simulink library "tools"  (R2015b)
settings: Solver=ode1  StartTime=0.0  StopTime=Inf  FixedStep=0.001  RelTol=1e-3
PostLoadFcn:
  | , if any(exist('dsrtsu_mdlpostloadfcn', 'file') == [2, 3, 6]), try dsrtsu_mdlpostloadfcn('Execute', bdroot); catch fprintf('Error in PostLoadFcn (dsrtsu_mdlpostloadfcn) for model "%s":\n %s\n', bdroot, lasterr); end, end,
libraries: tools x3, dspswit3 x2
settings Model: DSRTSU_INTERNAL_RTI_VER=460  DSRTSU_INTERNAL_RTI_TYPE=rti1401  DSRTSU_INTERNAL_RTIFPGA=50  Creator=luis  LastModifiedBy=luis
settings OptimizationCC: BlockReduction=off  OptimizeBlockIOStorage=off  BufferReuse=off  GlobalBufferReuse=off  ExpressionFolding=off  LocalBlockOutputs=off
settings HardwareCC: ProdEndianess=BigEndian  ProdWordSize=32  ProdHWDeviceType=Generic->Custom  TargetIntDivRoundTo=Zero  TargetEndianess=BigEndian  TargetHWDeviceType=Generic->Custom
settings RTWCC: SystemTargetFile=rti1401.tlc  MakeCommand=make_rti  TemplateMakefile=rti1401.tmf  Description=dSPACE DS1401 Hardware Platform
settings STFCustomTargetCC: ParMdlRefBuildCompliant=on  ConcurrentExecutionCompliant=off  GeneratePreprocessorConditionals=Use local settings  MatFileLogging=on  CPPClassGenCompliant=off  SystemTargetFile=rti1401.tlc
settings GRTTargetCC: CompOptLevelCompliant=off  ConcurrentExecutionCompliant=off  CombineOutputUpdateFcns=off  CPPClassGenCompliant=off  GRTInterface=on  UseToolchainInfoCompliant=off  ExtModeMexFile=noextcomm

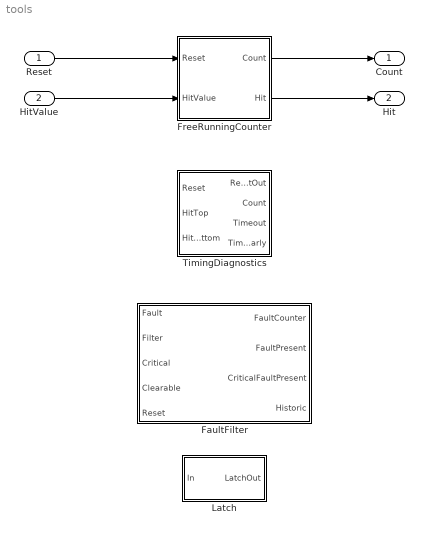
== system tools ==
  Reset : Inport
  HitValue : Inport  Port=2
  FaultFilter : Subsystem
  FreeRunningCounter : Subsystem
  Latch : Subsystem
  TimingDiagnostics : Subsystem
  Count : Outport
  Hit : Outport  Port=2
  wires:
  Reset/1 -> FreeRunningCounter/1(Reset)
  HitValue/1 -> FreeRunningCounter/2(HitValue)
  FreeRunningCounter/1(Count) -> Count/1
  FreeRunningCounter/2(Hit) -> Hit/1

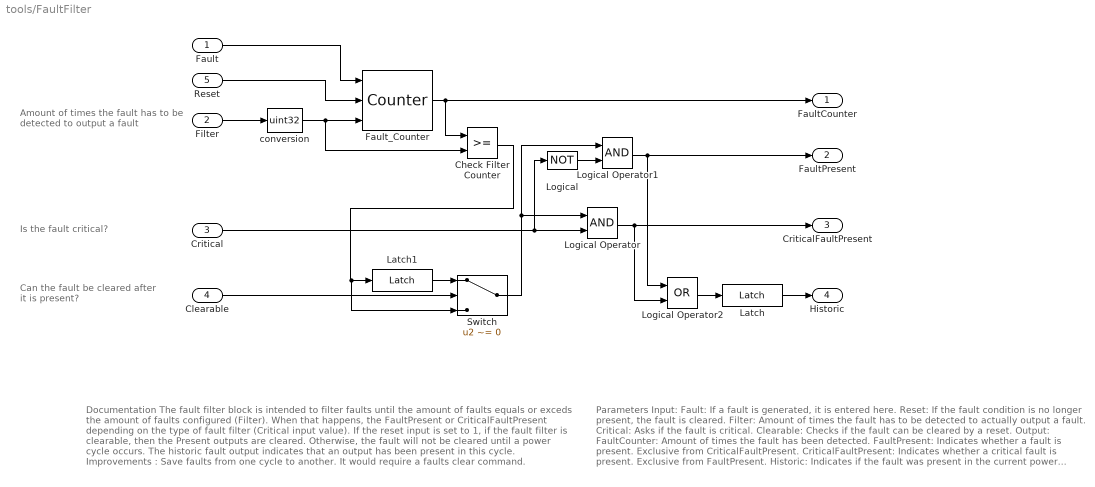
== system tools/FaultFilter ==
  note: Parameters
      | Input:
      | Fault: If a fault is generated, it is entered here.
      | Reset: If the fault condition is no longer present, the fault is cleared.
      | Filter: Amount of times the fault has to be detected to actually output a fault.
      | Critical: Asks if the fault is critical.
      | Clearable: Checks if the fault can be cleared by a reset.
      |
      | Output:
      | FaultCounter: Amount of times the fault has been detected.
      | FaultPresent: Indicates whether a fault is present. Exclusive from CriticalFaultPresent.
      | CriticalFaultPresent: Indicates whether a critical fault is present. Exclusive from FaultPresent.
      | Historic: Indicates if the fault was present in the current power cycle.
  note: Can the fault be cleared
      | after it is present?
  note: Is the fault critical?
  note: Amount of times the fault
      | has to be detected to output a fault
  note: Documentation
      | The fault filter block is intended to filter faults until the amount of faults equals or exceds the amount of faults configured (Filter). When that happens, the FaultPresent or CriticalFaultPresent depending on the type of fault filter (Critical input value). If the reset input is set to 1, if the fault filter is clearable, then the Present outputs are cleared.
      | Otherwise, the fault will not be cleared until a power cycle occurs.
      | The historic fault output indicates that an output has been present in this cycle.
      | Improvements : Save faults from one cycle to another. It would require a faults clear command.
  Fault : Inport
  Filter : Inport  Port=2
  Critical : Inport  Port=3
  Clearable : Inport  Port=4
  Reset : Inport  Port=5
  Check Filter Counter : RelationalOperator  OutDataTypeStr=boolean
  Fault_Counter : dspswit3/Counter  Direction=Up  CountEvent=Rising edge  CounterSize=Specify via input port  MaxCount=255  InitialCount=0  Output=Count  HitValue=32  ResetInput=on  SamplesPerFrame=1  Ts=-1  CntDtype=double  HitDtype=Logical
  Latch : tools/Latch
  Latch1 : tools/Latch
  Logical : Logic  Operator=NOT  AllPortsSameDT=off  OutDataTypeStr=boolean
  Logical Operator : Logic  AllPortsSameDT=off  OutDataTypeStr=boolean
  Logical Operator1 : Logic  AllPortsSameDT=off  OutDataTypeStr=boolean
  Logical Operator2 : Logic  Operator=OR  AllPortsSameDT=off  OutDataTypeStr=boolean
  Switch : Switch  Criteria=u2 ~= 0
  conversion : DataTypeConversion  OutDataTypeStr=uint32
  FaultCounter : Outport
  FaultPresent : Outport  Port=2
  CriticalFaultPresent : Outport  Port=3
  Historic : Outport  Port=4
  wires:
  Filter/1 -> conversion/1
  conversion/1 -> Fault_Counter/3, Check Filter Counter/2
  Reset/1 -> Fault_Counter/2
  Fault/1 -> Fault_Counter/1
  Latch/1 -> Historic/1
  Fault_Counter/1 -> FaultCounter/1, Check Filter Counter/1
  Critical/1 -> Logical/1, Logical Operator/2
  Logical Operator/1 -> Logical Operator2/2, CriticalFaultPresent/1
  Logical Operator1/1 -> FaultPresent/1, Logical Operator2/1
  Logical/1 -> Logical Operator1/2
  Logical Operator2/1 -> Latch/1
  Clearable/1 -> Switch/2
  Switch/1 -> Logical Operator/1, Logical Operator1/1
  Check Filter Counter/1 -> Switch/3, Latch1/1
  Latch1/1 -> Switch/1

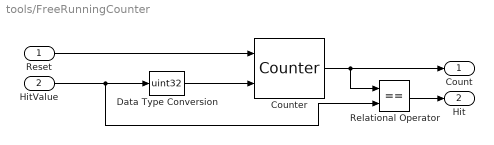
== system tools/FreeRunningCounter ==
  Reset : Inport
  HitValue : Inport  Port=2
  Counter : dspswit3/Counter  Direction=Up  CountEvent=Free running  CounterSize=Specify via input port  MaxCount=255  InitialCount=0  Output=Count  HitValue=32  ResetInput=on  SamplesPerFrame=1  Ts=-1  CntDtype=double  HitDtype=Logical
  Data Type Conversion : DataTypeConversion  OutDataTypeStr=uint32
  Relational Operator : RelationalOperator  Operator===  OutDataTypeStr=boolean
  Count : Outport
  Hit : Outport  Port=2
  wires:
  Data Type Conversion/1 -> Counter/2
  HitValue/1 -> Relational Operator/2, Data Type Conversion/1
  Counter/1 -> Relational Operator/1, Count/1
  Reset/1 -> Counter/1
  Relational Operator/1 -> Hit/1

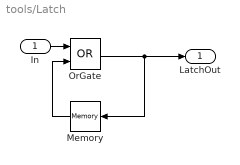
== system tools/Latch ==
  In : Inport
  Memory : Memory
  OrGate : Logic  Operator=OR  AllPortsSameDT=off  OutDataTypeStr=boolean
  LatchOut : Outport
  wires:
  Memory/1 -> OrGate/2
  In/1 -> OrGate/1
  OrGate/1 -> Memory/1, LatchOut/1

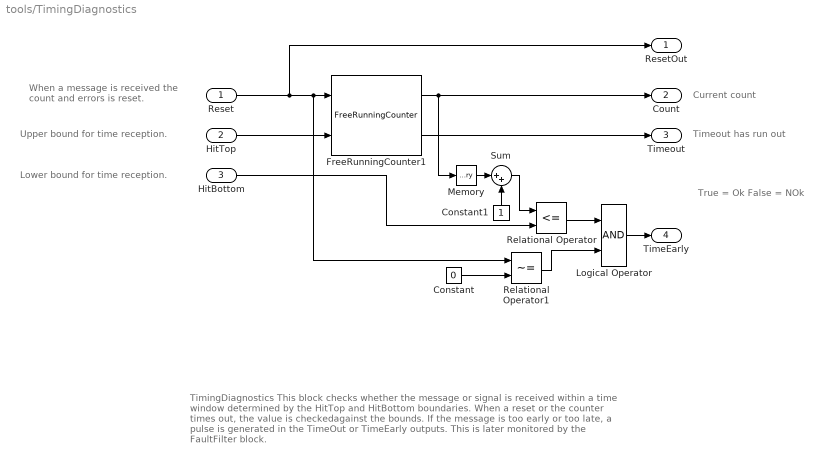
== system tools/TimingDiagnostics ==
  note: TimingDiagnostics
      | This block checks whether the message or signal is received within a time window determined by the HitTop and HitBottom boundaries.
      | When a reset or the counter times out, the value is checkedagainst the bounds. If the message is too early or too late, a pulse is generated in the TimeOut or TimeEarly outputs.
      | This is later monitored by the FaultFilter block.
  note: Upper bound for time reception.
  note: When a message is received
      | the count and errors is reset.
  note: Timeout has run out
  note: Current count
  note: True = Ok
      | False = NOk
  note: Lower bound for time reception.
  Reset : Inport
  HitTop : Inport  Port=2
  HitBottom : Inport  Port=3
  Constant : Constant  Value=0
  Constant1 : Constant
  FreeRunningCounter1 : tools/FreeRunningCounter
  Logical Operator : Logic  AllPortsSameDT=off  OutDataTypeStr=boolean
  Memory : Memory
  Relational Operator : RelationalOperator  Operator=<=  OutDataTypeStr=boolean
  Relational Operator1 : RelationalOperator  Operator=~=  OutDataTypeStr=boolean
  Sum : Sum  Inputs=|++
  ResetOut : Outport
  Count : Outport  Port=2
  Timeout : Outport  Port=3
  TimeEarly : Outport  Port=4
  wires:
  Constant1/1 -> Sum/2
  Memory/1 -> Sum/1
  Sum/1 -> Relational Operator/1
  Relational Operator1/1 -> Logical Operator/2
  Relational Operator/1 -> Logical Operator/1
  Constant/1 -> Relational Operator1/2
  Logical Operator/1 -> TimeEarly/1
  HitBottom/1 -> Relational Operator/2
  FreeRunningCounter1/1 -> Count/1, Memory/1
  HitTop/1 -> FreeRunningCounter1/2
  Reset/1 -> ResetOut/1, FreeRunningCounter1/1, Relational Operator1/1
  FreeRunningCounter1/2 -> Timeout/1
